simulink model "ThreeTankOpensystem"  (R2024a)
settings: Solver=VariableStepAuto  StartTime=0.0  StopTime=10.0  RelTol=1e-3
values from neighbouring files (symbols this model uses):
  A = [-f1 f1 0; f1 -2*f1 f1; 0 f1 -(f1+f2)]    [init_three_tank.m]
  Atank = pi*0.07^2    (= 0.0153938040026)    [init_three_tank.m]
  B = 1/Atank*[1 0; 0 0; 0 1]    [init_three_tank.m]
  g = 9.8    [init_three_tank.m]
  H = 0.1    [init_three_tank.m]
  href = [0.5; 0.4; 0.3]    [init_three_tank.m]
  q11 = q1ref*1.1    [init_three_tank.m]
  q1ref = Atube*sqrt(2*g*dh)    [init_three_tank.m]
  q21 = q2ref*0.9    [init_three_tank.m]
  q2ref = Atube*(-sqrt(2*g*dh)+sqrt(2*g*(href(3)-H)))    [init_three_tank.m]
  Ts = 0.1    [init_three_tank.m]
  tUnit = 60    [init_three_tank.m]
undefined symbols (not defined in the file or in its folder): DiscIntNeverNeededParam
settings Model: Creator=Aswathi C T  LastModifiedBy=Aswathi C T

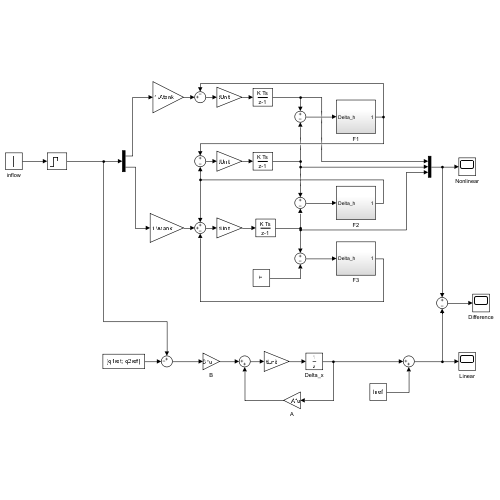
[thumbnail: Simulink's stored preview of the top-level diagram]
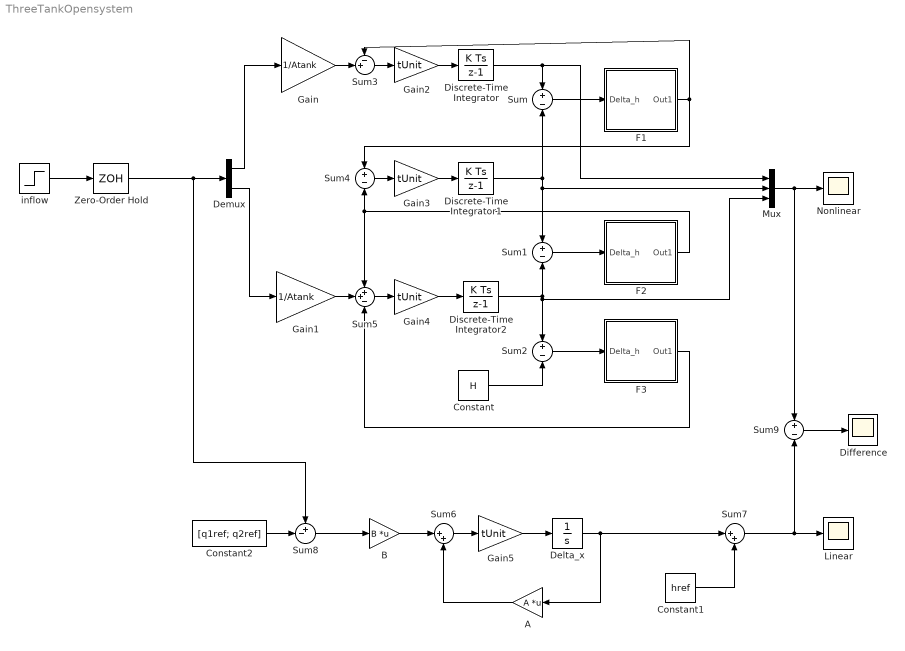
== system ThreeTankOpensystem ==
  A : Gain  Gain=A  Multiplication=Matrix(K*u)
  B : Gain  Gain=B  Multiplication=Matrix(K*u)
  Constant : Constant  Value=H
  Constant1 : Constant  Value=href
  Constant2 : Constant  Value=[q1ref; q2ref]
  Delta_x : Integrator  InitialCondition=[ 0; 0; 0 ]
  Demux : Demux  Outputs=2
  Difference : Scope
  Discrete-Time Integrator : DiscreteIntegrator  InitialCondition=0.5  SampleTime=Ts  ICPrevOutput=DiscIntNeverNeededParam  ICPrevScaledInput=DiscIntNeverNeededParam
  Discrete-Time Integrator1 : DiscreteIntegrator  InitialCondition=0.4  SampleTime=Ts  ICPrevOutput=DiscIntNeverNeededParam  ICPrevScaledInput=DiscIntNeverNeededParam
  Discrete-Time Integrator2 : DiscreteIntegrator  InitialCondition=0.3  SampleTime=Ts  ICPrevOutput=DiscIntNeverNeededParam  ICPrevScaledInput=DiscIntNeverNeededParam
  F1 : Subsystem
  F2 : Subsystem
  F3 : Subsystem
  Gain : Gain  Gain=1/Atank
  Gain1 : Gain  Gain=1/Atank
  Gain{2..5} (4 alike) : Gain  Gain=tUnit
  Linear : Scope
  Mux : Mux  Inputs=3
  Nonlinear : Scope
  Sum{,1..2,4,9} (5 alike) : Sum  Inputs=+-
  Sum3 : Sum  Inputs=-+|
  Sum5 : Sum  Inputs=++-
  Sum6 : Sum  Inputs=|++
  Sum7 : Sum  Inputs=|++
  Sum8 : Sum  Inputs=+-|
  Zero-Order Hold : ZeroOrderHold  SampleTime=-1
  inflow : Step  Before=[q1ref;q2ref]  After=[q11;q21]  SampleTime=0
  wires:
  Gain4/1 -> Discrete-Time Integrator2/1
  Gain5/1 -> Delta_x/1
  Sum9/1 -> Difference/1
  Delta_x/1 -> Sum7/1, A/1
  F1/1(Out1) -> Sum4/1, Sum3/1
  Sum6/1 -> Gain5/1
  Demux/1 -> Gain/1
  Gain3/1 -> Discrete-Time Integrator1/1
  Sum8/1 -> B/1
  Gain2/1 -> Discrete-Time Integrator/1
  inflow/1 -> Zero-Order Hold/1
  Discrete-Time Integrator/1 -> Mux/1, Sum/1
  Constant1/1 -> Sum7/2
  Constant2/1 -> Sum8/2
  A/1 -> Sum6/2
  F2/1(Out1) -> Sum4/2, Sum5/1
  Sum5/1 -> Gain4/1
  Mux/1 -> Sum9/1, Nonlinear/1
  B/1 -> Sum6/1
  F3/1(Out1) -> Sum5/3
  Sum1/1 -> F2/1(Delta_h)
  Sum2/1 -> F3/1(Delta_h)
  Discrete-Time Integrator2/1 -> Sum1/2, Mux/3, Sum2/1
  Sum7/1 -> Sum9/2, Linear/1
  Demux/2 -> Gain1/1
  Sum/1 -> F1/1(Delta_h)
  Gain/1 -> Sum3/2
  Gain1/1 -> Sum5/2
  Sum3/1 -> Gain2/1
  Constant/1 -> Sum2/2
  Sum4/1 -> Gain3/1
  Discrete-Time Integrator1/1 -> Sum1/1, Mux/2, Sum/2
  Zero-Order Hold/1 -> Sum8/1, Demux/1

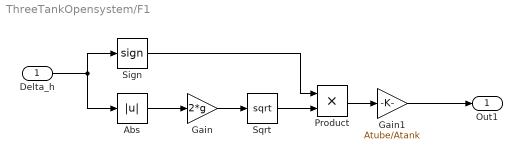
== system ThreeTankOpensystem/F1 ==
  Delta_h : Inport
  Abs : Abs  SaturateOnIntegerOverflow=off
  Gain : Gain  Gain=2*g
  Gain1 : Gain  Gain=Atube/Atank
  Product : Product
  Sign : Signum
  Sqrt : Sqrt
  Out1 : Outport
  wires:
  Product/1 -> Gain1/1
  Gain1/1 -> Out1/1
  Sign/1 -> Product/1
  Sqrt/1 -> Product/2
  Delta_h/1 -> Abs/1, Sign/1
  Abs/1 -> Gain/1
  Gain/1 -> Sqrt/1

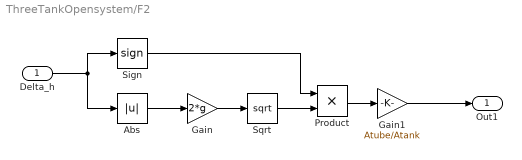
== system ThreeTankOpensystem/F2 ==
  Delta_h : Inport
  Abs : Abs  SaturateOnIntegerOverflow=off
  Gain : Gain  Gain=2*g
  Gain1 : Gain  Gain=Atube/Atank
  Product : Product
  Sign : Signum
  Sqrt : Sqrt
  Out1 : Outport
  wires:
  Gain/1 -> Sqrt/1
  Abs/1 -> Gain/1
  Delta_h/1 -> Sign/1, Abs/1
  Sqrt/1 -> Product/2
  Sign/1 -> Product/1
  Gain1/1 -> Out1/1
  Product/1 -> Gain1/1

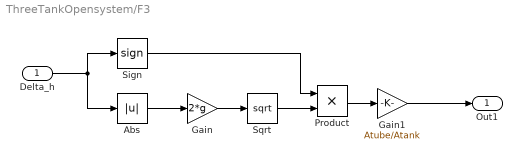
== system ThreeTankOpensystem/F3 ==
  Delta_h : Inport
  Abs : Abs  SaturateOnIntegerOverflow=off
  Gain : Gain  Gain=2*g
  Gain1 : Gain  Gain=Atube/Atank
  Product : Product
  Sign : Signum
  Sqrt : Sqrt
  Out1 : Outport
  wires:
  Product/1 -> Gain1/1
  Gain1/1 -> Out1/1
  Sign/1 -> Product/1
  Sqrt/1 -> Product/2
  Delta_h/1 -> Abs/1, Sign/1
  Abs/1 -> Gain/1
  Gain/1 -> Sqrt/1
